simulink model "MC_Phase2_Part1_Q3_Sim_v3"  (R2020b)
settings: Solver=VariableStepAuto  StartTime=0.0  StopTime=10.0  RelTol=1e-3
settings Model: Creator=1007  LastModifiedBy=1007

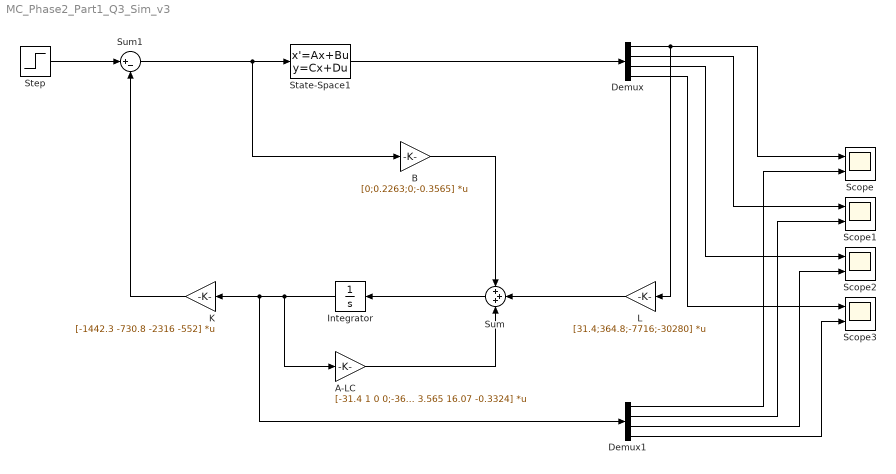
== system MC_Phase2_Part1_Q3_Sim_v3 ==
  A-LC : Gain  Gain=[-31.4 1 0 0;-364.8 -2.263 -0.3963 0.0082; 7716 0 0 1; 30280 3.565 16.07 -0.3324]  Multiplication=Matrix(K*u)
  B : Gain  Gain=[0;0.2263;0;-0.3565]  Multiplication=Matrix(K*u)
  Demux : Demux
  Demux1 : Demux
  Integrator : Integrator
  K : Gain  Gain=[-1442.3 -730.8 -2316 -552]  Multiplication=Matrix(K*u)
  L : Gain  Gain=[31.4;364.8;-7716;-30280]  Multiplication=Matrix(K*u)
  Scope{,1..3} (4 alike) : Scope  NumInputPorts=2
  State-Space1 : StateSpace  A=[0 1 0 0;0 -2.2626 -0.3963 0.0082;0 0 0 1;0 3.5649 16.0655 -0.3324]  B=[0 ;0.2263 ;0 ;-0.3565 ]  C=[1 0 0 0;0 1 0 0;0 0 1 0;0 0 0 1]  D=[0;0;0;0]  InitialCondition=0
  Step : Step  SampleTime=0
  Sum : Sum  Inputs=+++
  Sum1 : Sum  Inputs=|+-
  wires:
  L/1 -> Sum/2
  Sum/1 -> Integrator/1
  B/1 -> Sum/1
  Integrator/1 -> Demux1/1, K/1, A-LC/1
  A-LC/1 -> Sum/3
  Step/1 -> Sum1/1
  Sum1/1 -> B/1, State-Space1/1
  K/1 -> Sum1/2
  State-Space1/1 -> Demux/1
  Demux/1 -> L/1, Scope/1
  Demux1/1 -> Scope/2
  Demux/2 -> Scope1/1
  Demux1/2 -> Scope1/2
  Demux/3 -> Scope2/1
  Demux/4 -> Scope3/1
  Demux1/3 -> Scope2/2
  Demux1/4 -> Scope3/2
